simulink model "APFC_FullModel_v21b_Qmeas"  (R2025b)
settings: Solver=ode23t  StartTime=0.0  StopTime=50  MaxStep=2e-4  RelTol=1e-3
undefined symbols (not defined in the file): a_dq, ALPF_FAP_a, ALPF_FAP_b, ALPF_fine_alpha_delta, ALPF_fs, ALPF_gross_alpha, ALPF_k_powerOn, ALPF_LPF_g, ALPF_LPF_mag50_lin, ALPF_LPF_sos, ALPF_offset_inc_fine, ALPF_offset_inc_gross, b_dq, C_B1, C_B2, C_B3, DiscIntNeverNeededParam, dspblkCoreblockFVToolHelper, FLC_deadband_kVAR, gcbh, L_B1, L_B2, L_B3, omega, p, Q_reactor, Rc, tau_Qload, X1
libraries: ee_lib x63, fl_lib x59, nesl_utility x43, simulink x18, dspswit3 x9, dsparch4 x3, eeTransforms x2, fuzblock x1, eeSinusoidalMeasurementV2 x1
(part 2 of 5)

== system APFC_FullModel_v21b_Qmeas/ALPF2/CTRL ==
  IN : Inport
  YOUT : Inport  Port=2
  FSM : Subsystem  mask(ALPF CTRL FSM){}
      mask help:
      | ALPF CTRL FSM (Dossi US 12,294,375 B2, block 24). Parallel (AND) Stateflow
      | decomposition: phase branch ST0/ST1/ST2 on DIST, offset branch ST0/ST3/ST4 on
      | DISTORT, concurrent and independent. Three-threshold hysteresis per branch:
      | leave lock at |metric|>9, return at <3, escalate to gross at >21.
      | Phase: gross steps index by DIR and reads alpha = ALPF_gross_alpha(index); fine
      | accumulates alpha += ALPF_fine_alpha_delta(index)*DIR at the frozen index.
      | Offset: accumulates ADJ_offset by ALPF_offset_inc_fine (ST3) / ALPF_offset_inc_gross
      | (ST4), times the per-cycle OFFSET. Power-on index = ALPF_k_powerOn (40).
      | Reads ALPF_gross_alpha, ALPF_fine_alpha_delta, ALPF_k_powerOn, ALPF_offset_inc_fine,
      | ALPF_offset_inc_gross from the base workspace (APFC_Parameters.m). Double precision. Built and verified in four prove-then-mask stages. Documentation-only mask.
  OffsetBuffer : Subsystem  TreatAsAtomicUnit=on  mask(ALPF Phase Buffer){N=45}
      mask prompts: N "Buffer length N"
      mask help: FIFO of the most recent N=45 OFFSET values, clocked once per cycle by DZC; DISTORT = sum of buffer = distortion/offset metric, range −45…+45.
  PhaseBuffer : Subsystem  TreatAsAtomicUnit=on  mask(ALPF Phase Buffer){N=45}
      mask prompts: N "Buffer length N"
      mask help: FIFO of the most recent N=45 DIR values, clocked once per cycle by DZC; DIST = sum of buffer = phase‑mismatch metric, range −45…+45.
  SlopeDetector : Subsystem  mask(ALPF Slope Detector){}
      mask help: Computes SLOPE = |Slope_IN − Slope_YOUT| for the ALPF zero-crossing detector's adaptive threshold RESOL_THRES = MAX(IN)/4096 + SLOPE/4. Each per-sample slope (backward difference) is sampled and held at its own positive-going zero crossing. The absolute value guarantees SLOPE ≥ 0 so RESOL_THRES never falls below its MAX(IN)/4096 floor. Per Dossi patent (US 12,294,375 B2), block 21. SLOPE in per-sample units.
  ZCD : Subsystem  mask(ALPF Zero-Crossing Detector){}
      mask help: Computes zc=(IN+YOUT)/2; detects positive-going crossings of IN and YOUT; latches INC at YOUT's crossing and decodes DIR=INC−DEC, OFFSET=1−INC−DEC at IN's crossing (cycle boundary). RESOL_THRES = MAX(IN)/4096 + SLOPE/4.
  alpha : Outport
  index : Outport  Port=2
  ADJ_offset : Outport  Port=3
  SLOPE : Outport  Port=4
  DIR : Outport  Port=5
  DIST : Outport  Port=6
  OFFSET : Outport  Port=7
  DISTORT : Outport  Port=8
  wires:
  FSM/2(index) -> index/1
  ZCD/2(OFFSET) -> FSM/5(OFFSET), OFFSET/1, OffsetBuffer/1(OFFSET)  "OFFSET"
  ZCD/3(DZC) -> FSM/1(DZC), PhaseBuffer/Trigger, OffsetBuffer/Trigger
  IN/1 -> ZCD/1(IN), SlopeDetector/1(IN)
  YOUT/1 -> SlopeDetector/2(YOUT), ZCD/2(YOUT)
  ZCD/1(DIR) -> DIR/1, FSM/4(DIR), PhaseBuffer/1(DIR)  "DIR"
  SlopeDetector/1(SLOPE) -> SLOPE/1, ZCD/3(SLOPE)  "SLOPE"
  OffsetBuffer/1(DISTORT) -> FSM/3(DISTORT), DISTORT/1  "DISTORT"
  PhaseBuffer/1(DIST) -> DIST/1, FSM/2(DIST)  "DIST"
  FSM/1(alpha) -> alpha/1
  FSM/3(ADJ_offset) -> ADJ_offset/1

== system APFC_FullModel_v21b_Qmeas/ALPF2/FAP ==
  LPF_OUT : Inport
  Discrete Filter : DiscreteFilter  LoadFcn=dspblkCoreblockFVToolHelper(gcbh,'load');  Numerator=ALPF_FAP_b  Denominator=ALPF_FAP_a  FilterStructure=Direct form II transposed  a0EqualsOne=on
      settings: CopyFcn=dspblkCoreblockFVToolHelper(gcbh,'copy');  DeleteFcn=dspblkCoreblockFVToolHelper(gcbh,'close');  ModelCloseFcn=dspblkCoreblockFVToolHelper(gcbh,'close');  PreSaveFcn=dspblkCoreblockFVToolHelper(gcbh,'presave');  PostSaveFcn=dspblkCoreblockFVToolHelper(gcbh,'postsave');  CloseFcn=dspblkCoreblockFVToolHelper(gcbh,'close');
  FAP_OUT : Outport
  wires:
  LPF_OUT/1 -> Discrete Filter/1
  Discrete Filter/1 -> FAP_OUT/1

== system APFC_FullModel_v21b_Qmeas/ALPF2/LPF ==
  IN : Inport
  Biquad Filter : dsparch4/Biquad Filter  FilterSource=Dialog parameters  CoeffSource=Specify via dialog  FilterObject=BQF  IIRFiltStruct=Direct form II transposed  BiQuadCoeffs=ALPF_LPF_sos  ScaleValues=ALPF_LPF_g  IC=0  ICnum=0  ICden=0  a0Flag=Error  optimizeScaleValues=on  ScaleValueMode=Specify via input port (g)  roundingMode=Floor  overflowMode=off  scaleValueFracLength=14  denProdOutputFracLength=30  denAccumFracLength=30  secondMemoryFracLength=15
  LPF_OUT : Outport
  wires:
  Biquad Filter/1 -> LPF_OUT/1
  IN/1 -> Biquad Filter/1

== system APFC_FullModel_v21b_Qmeas/TSC Compensator/Bank_1 (5 kVAR) ==
  Enable_B1 : Inport
  TSC Bank 1 : Subsystem
      mask help:
      | Three-phase delta-connected TSC bank subsystem.
      | Contains three identical Delta_Limb instances (AB, BC, CA) and three line-to-line voltage sensors.
      |
      | Parameters C_val, L_val, and Rd_val are passed to all three Delta_Limb instances.
      | Default values correspond to Bank 1 (5 kVAR) at 415 V / 50 Hz with 6% detuning factor.
      |
      | Electrical ports: Phase_A, Phase_B, Phase_C.
      | Simulink inports: Gate_Drive_AB, Gate_Drive_BC, Gate_Drive_CA.
      | Simulink outports: V_AB, V_BC, V_CA (line voltages),
      | V_C0_AB, V_C0_BC, V_C0_CA (capacitor voltages),
      | V_sw_AB, V_sw_BC, V_sw_CA (thyristor switching voltages) are accessible via internal Scope blocks inside this subsystem.
      |
      | ZCD logic and Enable signals are external to this subsystem.
  ZCD Bank 1 : Subsystem
      mask help:
      | ZCD_Bank subsystem for one three-phase delta-connected TSC bank.
      | Contains ZCD_AB, ZCD_BC, ZCD_CA — one per delta limb.
      |
      | Inports: V_AB, V_BC, V_CA (line voltages from TSC_Bank),
      | V_C0_AB, V_C0_BC, V_C0_CA (capacitor voltages from TSC_Bank),
      | Enable (single switching command, broadcast to all three ZCDs).
      |
      | Outports: Gate_Drive_AB, Gate_Drive_BC, Gate_Drive_CA.
      |
      | One instance required per bank: ZCD_Bank_B1, ZCD_Bank_B2,
      | ZCD_Bank_B3.
  Phase_A : PMIOPort  Side=Left
  Phase_B : PMIOPort  Port=2  Side=Left
  Phase_C : PMIOPort  Port=3  Side=Left
  wires:
  TSC Bank 1/5(V_CA) -> ZCD Bank 1/5(V_CA)  "V_CA_B1"
  TSC Bank 1/2(V_CO_AB) -> ZCD Bank 1/2(V_CO_AB)  "V_CO_AB_B1"
  Enable_B1/1 -> ZCD Bank 1/7(Enable)
  TSC Bank 1/3(V_BC) -> ZCD Bank 1/3(V_BC)  "V_BC_B1"
  TSC Bank 1/1(V_AB) -> ZCD Bank 1/1(V_AB)  "V_AB_B1"
  TSC Bank 1/6(V_CO_CA) -> ZCD Bank 1/6(V_CO_CA)  "V_CO_CA_B1"
  TSC Bank 1/4(V_CO_BC) -> ZCD Bank 1/4(V_CO_BC)  "V_CO_BC_B1"
  ZCD Bank 1/1(Gate_drive_AB) -> TSC Bank 1/1(Gate_Drive_AB)
  ZCD Bank 1/2(Gate_drive_BC) -> TSC Bank 1/2(Gate_Drive_BC)
  ZCD Bank 1/3(Gate_drive_CA) -> TSC Bank 1/3(Gate_Drive_CA)
  connections:
  TSC Bank 1/LConn2 -- Phase_B/RConn1
  TSC Bank 1/LConn3 -- Phase_C/RConn1
  TSC Bank 1/LConn1 -- Phase_A/RConn1

== system APFC_FullModel_v21b_Qmeas/TSC Compensator/Bank_2 (10 kVAR) ==
  Enable_B2 : Inport
  TSC Bank 2 : Subsystem
      mask help:
      | Three-phase delta-connected TSC bank subsystem.
      | Contains three identical Delta_Limb instances (AB, BC, CA) and three line-to-line voltage sensors.
      |
      | Parameters C_val, L_val, and Rd_val are passed to all three Delta_Limb instances.
      | Default values correspond to Bank 2 (10 kVAR) at 415 V / 50 Hz with 6% detuning factor.
      |
      | Electrical ports: Phase_A, Phase_B, Phase_C.
      | Simulink inports: Gate_Drive_AB, Gate_Drive_BC, Gate_Drive_CA.
      | Simulink outports: V_AB, V_BC, V_CA (line voltages),
      | V_C0_AB, V_C0_BC, V_C0_CA (capacitor voltages),
      | V_sw_AB, V_sw_BC, V_sw_CA (thyristor switching voltages) are accessible via internal Scope blocks inside this subsystem.
      |
      | ZCD logic and Enable signals are external to this subsystem.
  ZCD Bank 2 : Subsystem
      mask help:
      | ZCD_Bank subsystem for one three-phase delta-connected TSC bank.
      | Contains ZCD_AB, ZCD_BC, ZCD_CA — one per delta limb.
      |
      | Inports: V_AB, V_BC, V_CA (line voltages from TSC_Bank),
      | V_C0_AB, V_C0_BC, V_C0_CA (capacitor voltages from TSC_Bank),
      | Enable (single switching command, broadcast to all three ZCDs).
      |
      | Outports: Gate_Drive_AB, Gate_Drive_BC, Gate_Drive_CA.
      |
      | One instance required per bank: ZCD_Bank_B1, ZCD_Bank_B2,
      | ZCD_Bank_B3.
  Phase_A : PMIOPort  Side=Left
  Phase_B : PMIOPort  Port=2  Side=Left
  Phase_C : PMIOPort  Port=3  Side=Left
  wires:
  TSC Bank 2/2(V_CO_AB) -> ZCD Bank 2/2(V_CO_AB)  "V_CO_AB_B2"
  TSC Bank 2/6(V_CO_CA) -> ZCD Bank 2/6(V_CO_CA)  "V_CO_CA_B2"
  TSC Bank 2/3(V_BC) -> ZCD Bank 2/3(V_BC)  "V_BC_B2"
  TSC Bank 2/5(V_CA) -> ZCD Bank 2/5(V_CA)  "V_CA_B2"
  TSC Bank 2/1(V_AB) -> ZCD Bank 2/1(V_AB)  "V_AB_B2"
  TSC Bank 2/4(V_CO_BC) -> ZCD Bank 2/4(V_CO_BC)  "V_CO_BC_B2"
  Enable_B2/1 -> ZCD Bank 2/7(Enable)
  ZCD Bank 2/1(Gate_drive_AB) -> TSC Bank 2/1(Gate_Drive_AB)
  ZCD Bank 2/2(Gate_drive_BC) -> TSC Bank 2/2(Gate_Drive_BC)
  ZCD Bank 2/3(Gate_drive_CA) -> TSC Bank 2/3(Gate_Drive_CA)
  connections:
  TSC Bank 2/LConn1 -- Phase_A/RConn1
  TSC Bank 2/LConn2 -- Phase_B/RConn1
  TSC Bank 2/LConn3 -- Phase_C/RConn1

== system APFC_FullModel_v21b_Qmeas/TSC Compensator/Bank_3 (20 kVAR) ==
  Enable_B3 : Inport
  TSC Bank 3 : Subsystem
      mask help:
      | Three-phase delta-connected TSC bank subsystem.
      | Contains three identical Delta_Limb instances (AB, BC, CA) and three line-to-line voltage sensors.
      |
      | Parameters C_val, L_val, and Rd_val are passed to all three Delta_Limb instances.
      | Default values correspond to Bank 3 (20 kVAR) at 415 V / 50 Hz with 6% detuning factor.
      |
      | Electrical ports: Phase_A, Phase_B, Phase_C.
      | Simulink inports: Gate_Drive_AB, Gate_Drive_BC, Gate_Drive_CA.
      | Simulink outports: V_AB, V_BC, V_CA (line voltages),
      | V_C0_AB, V_C0_BC, V_C0_CA (capacitor voltages),
      | V_sw_AB, V_sw_BC, V_sw_CA (thyristor switching voltages) are accessible via internal Scope blocks inside this subsystem.
      |
      | ZCD logic and Enable signals are external to this subsystem.
  ZCD Bank 3 : Subsystem
      mask help:
      | ZCD_Bank subsystem for one three-phase delta-connected TSC bank.
      | Contains ZCD_AB, ZCD_BC, ZCD_CA — one per delta limb.
      |
      | Inports: V_AB, V_BC, V_CA (line voltages from TSC_Bank),
      | V_C0_AB, V_C0_BC, V_C0_CA (capacitor voltages from TSC_Bank),
      | Enable (single switching command, broadcast to all three ZCDs).
      |
      | Outports: Gate_Drive_AB, Gate_Drive_BC, Gate_Drive_CA.
      |
      | One instance required per bank: ZCD_Bank_B1, ZCD_Bank_B2,
      | ZCD_Bank_B3.
  Phase_A : PMIOPort  Side=Left
  Phase_B : PMIOPort  Port=2  Side=Left
  Phase_C : PMIOPort  Port=3  Side=Left
  wires:
  TSC Bank 3/3(V_BC) -> ZCD Bank 3/3(V_BC)  "V_BC_B3"
  TSC Bank 3/4(V_CO_BC) -> ZCD Bank 3/4(V_CO_BC)  "V_CO_BC_B3"
  TSC Bank 3/6(V_CO_CA) -> ZCD Bank 3/6(V_CO_CA)  "V_CO_CA_B3"
  TSC Bank 3/5(V_CA) -> ZCD Bank 3/5(V_CA)  "V_CA_B3"
  TSC Bank 3/2(V_CO_AB) -> ZCD Bank 3/2(V_CO_AB)  "V_CO_AB_B3"
  TSC Bank 3/1(V_AB) -> ZCD Bank 3/1(V_AB)  "V_AB_B3"
  Enable_B3/1 -> ZCD Bank 3/7(Enable)
  ZCD Bank 3/1(Gate_drive_AB) -> TSC Bank 3/1(Gate_Drive_AB)
  ZCD Bank 3/2(Gate_drive_BC) -> TSC Bank 3/2(Gate_Drive_BC)
  ZCD Bank 3/3(Gate_drive_CA) -> TSC Bank 3/3(Gate_Drive_CA)
  connections:
  Phase_B/RConn1 -- TSC Bank 3/LConn2
  Phase_A/RConn1 -- TSC Bank 3/LConn1
  Phase_C/RConn1 -- TSC Bank 3/LConn3

== system APFC_FullModel_v21b_Qmeas/ALPF/CTRL/FSM ==
  DZC : Inport
  DIST : Inport  Port=2
  DISTORT : Inport  Port=3
  DIR : Inport  Port=4
  OFFSET : Inport  Port=5
  ALPF_FSM : Stateflow chart  TreatAsAtomicUnit=on
  alpha : Outport
  index : Outport  Port=2
  ADJ_offset : Outport  Port=3
  wires:
  ALPF_FSM/2(index) -> index/1
  DZC/1 -> ALPF_FSM/Trigger
  OFFSET/1 -> ALPF_FSM/4(OFFSET)
  ALPF_FSM/1(alpha) -> alpha/1
  DISTORT/1 -> ALPF_FSM/2(DISTORT)
  ALPF_FSM/3(ADJ_offset) -> ADJ_offset/1
  DIST/1 -> ALPF_FSM/1(DIST)
  DIR/1 -> ALPF_FSM/3(DIR)

== system APFC_FullModel_v21b_Qmeas/ALPF/CTRL/OffsetBuffer ==
  OFFSET : Inport
  Trigger : TriggerPort  VariantControl=(inherit)
  Sum of Elements : Sum  Inputs=+
  Tapped Delay : simulink/Discrete/Tapped Delay  vinit=0.0  samptime=-1  NumDelays=N-1  DelayOrder=Oldest  includeCurrent=on
  DISTORT : Outport
  wires:
  OFFSET/1 -> Tapped Delay/1
  Tapped Delay/1 -> Sum of Elements/1
  Sum of Elements/1 -> DISTORT/1

== system APFC_FullModel_v21b_Qmeas/ALPF/CTRL/PhaseBuffer ==
  DIR : Inport
  Trigger : TriggerPort  VariantControl=(inherit)
  Sum of Elements : Sum  Inputs=+
  Tapped Delay : simulink/Discrete/Tapped Delay  vinit=0.0  samptime=-1  NumDelays=N-1  DelayOrder=Oldest  includeCurrent=on
  DIST : Outport
  wires:
  DIR/1 -> Tapped Delay/1
  Tapped Delay/1 -> Sum of Elements/1
  Sum of Elements/1 -> DIST/1

== system APFC_FullModel_v21b_Qmeas/ALPF/CTRL/SlopeDetector ==
  IN : Inport
  YOUT : Inport  Port=2
  Abs : Abs  SaturateOnIntegerOverflow=off
  Detect Rise Nonnegative : simulink/Logic and Bit Operations/Detect Rise Nonnegative  vinit=0  OutDataTypeStr=boolean
  Detect Rise Nonnegative1 : simulink/Logic and Bit Operations/Detect Rise Nonnegative  vinit=0  OutDataTypeStr=boolean
  Hold_SlopeIN : Subsystem  TreatAsAtomicUnit=on
  Hold_SlopeYOUT : Subsystem  TreatAsAtomicUnit=on
  Subtract : Sum  Inputs=+-
  Subtract1 : Sum  Inputs=+-
  Subtract2 : Sum  Inputs=+-
  Unit Delay : UnitDelay  SampleTime=1/12500  HasFrameUpgradeWarning=on
  Unit Delay1 : UnitDelay  SampleTime=1/12500  HasFrameUpgradeWarning=on
  SLOPE : Outport
  wires:
  Subtract2/1 -> Abs/1  "Slope_diff"
  Abs/1 -> SLOPE/1  "SLOPE"
  Hold_SlopeYOUT/1(Out1) -> Subtract2/2  "Slope_YOUT_held"
  YOUT/1 -> Detect Rise Nonnegative1/1, Unit Delay1/1, Subtract1/1
  Detect Rise Nonnegative/1 -> Hold_SlopeIN/Trigger  "IN_posZC"
  Subtract/1 -> Hold_SlopeIN/1(In1)  "Slope_IN"
  Unit Delay1/1 -> Subtract1/2
  Detect Rise Nonnegative1/1 -> Hold_SlopeYOUT/Trigger  "YOUT_posZC"
  IN/1 -> Unit Delay/1, Detect Rise Nonnegative/1, Subtract/1
  Subtract1/1 -> Hold_SlopeYOUT/1(In1)  "Slope_YOUT"
  Hold_SlopeIN/1(Out1) -> Subtract2/1  "Slope_IN_held"
  Unit Delay/1 -> Subtract/2

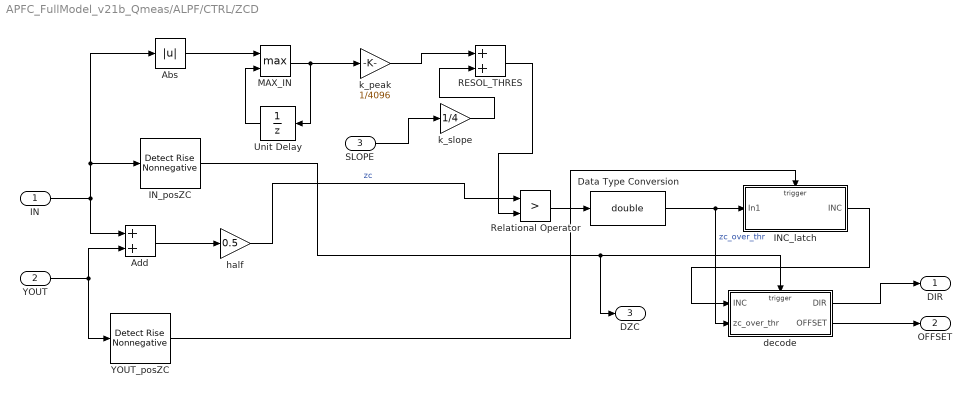
== system APFC_FullModel_v21b_Qmeas/ALPF/CTRL/ZCD ==
  IN : Inport
  YOUT : Inport  Port=2
  SLOPE : Inport  Port=3
  Abs : Abs  SaturateOnIntegerOverflow=off
  Add : Sum
  Data Type Conversion : DataTypeConversion  OutDataTypeStr=double  SaturateOnIntegerOverflow=off  RndMeth=Floor
  INC_latch : Subsystem  TreatAsAtomicUnit=on
  IN_posZC : simulink/Logic and Bit Operations/Detect Rise Nonnegative  vinit=0  OutDataTypeStr=boolean
  MAX_IN : MinMax  Function=max  Inputs=2
  RESOL_THRES : Sum
  Relational Operator : RelationalOperator  Operator=>  OutDataTypeStr=boolean  RndMeth=Simplest  InputSameDT=off
  Unit Delay : UnitDelay  SampleTime=1/12500  HasFrameUpgradeWarning=on
  YOUT_posZC : simulink/Logic and Bit Operations/Detect Rise Nonnegative  vinit=0  OutDataTypeStr=boolean
  decode : Subsystem  TreatAsAtomicUnit=on
  half : Gain  Gain=0.5
  k_peak : Gain  Gain=1/4096
  k_slope : Gain  Gain=1/4
  DIR : Outport
  OFFSET : Outport  Port=2
  DZC : Outport  Port=3
  wires:
  Data Type Conversion/1 -> decode/2(zc_over_thr), INC_latch/1(In1)  "zc_over_thr"
  half/1 -> Relational Operator/1  "zc"
  Relational Operator/1 -> Data Type Conversion/1
  SLOPE/1 -> k_slope/1
  YOUT/1 -> YOUT_posZC/1, Add/2
  RESOL_THRES/1 -> Relational Operator/2
  Add/1 -> half/1
  decode/1(DIR) -> DIR/1
  IN/1 -> IN_posZC/1, Abs/1, Add/1
  YOUT_posZC/1 -> INC_latch/Trigger
  MAX_IN/1 -> Unit Delay/1, k_peak/1
  IN_posZC/1 -> DZC/1, decode/Trigger
  INC_latch/1(INC) -> decode/1(INC)
  Unit Delay/1 -> MAX_IN/2
  Abs/1 -> MAX_IN/1
  k_slope/1 -> RESOL_THRES/2
  decode/2(OFFSET) -> OFFSET/1
  k_peak/1 -> RESOL_THRES/1

== system APFC_FullModel_v21b_Qmeas/ALPF1/CTRL/FSM ==
  DZC : Inport
  DIST : Inport  Port=2
  DISTORT : Inport  Port=3
  DIR : Inport  Port=4
  OFFSET : Inport  Port=5
  ALPF_FSM : Stateflow chart  TreatAsAtomicUnit=on
  alpha : Outport
  index : Outport  Port=2
  ADJ_offset : Outport  Port=3
  wires:
  ALPF_FSM/2(index) -> index/1
  DZC/1 -> ALPF_FSM/Trigger
  OFFSET/1 -> ALPF_FSM/4(OFFSET)
  ALPF_FSM/1(alpha) -> alpha/1
  DISTORT/1 -> ALPF_FSM/2(DISTORT)
  ALPF_FSM/3(ADJ_offset) -> ADJ_offset/1
  DIST/1 -> ALPF_FSM/1(DIST)
  DIR/1 -> ALPF_FSM/3(DIR)

== system APFC_FullModel_v21b_Qmeas/ALPF1/CTRL/OffsetBuffer ==
  OFFSET : Inport
  Trigger : TriggerPort  VariantControl=(inherit)
  Sum of Elements : Sum  Inputs=+
  Tapped Delay : simulink/Discrete/Tapped Delay  vinit=0.0  samptime=-1  NumDelays=N-1  DelayOrder=Oldest  includeCurrent=on
  DISTORT : Outport
  wires:
  OFFSET/1 -> Tapped Delay/1
  Tapped Delay/1 -> Sum of Elements/1
  Sum of Elements/1 -> DISTORT/1

== system APFC_FullModel_v21b_Qmeas/ALPF1/CTRL/PhaseBuffer ==
  DIR : Inport
  Trigger : TriggerPort  VariantControl=(inherit)
  Sum of Elements : Sum  Inputs=+
  Tapped Delay : simulink/Discrete/Tapped Delay  vinit=0.0  samptime=-1  NumDelays=N-1  DelayOrder=Oldest  includeCurrent=on
  DIST : Outport
  wires:
  DIR/1 -> Tapped Delay/1
  Tapped Delay/1 -> Sum of Elements/1
  Sum of Elements/1 -> DIST/1

== system APFC_FullModel_v21b_Qmeas/ALPF1/CTRL/SlopeDetector ==
  IN : Inport
  YOUT : Inport  Port=2
  Abs : Abs  SaturateOnIntegerOverflow=off
  Detect Rise Nonnegative : simulink/Logic and Bit Operations/Detect Rise Nonnegative  vinit=0  OutDataTypeStr=boolean
  Detect Rise Nonnegative1 : simulink/Logic and Bit Operations/Detect Rise Nonnegative  vinit=0  OutDataTypeStr=boolean
  Hold_SlopeIN : Subsystem  TreatAsAtomicUnit=on
  Hold_SlopeYOUT : Subsystem  TreatAsAtomicUnit=on
  Subtract : Sum  Inputs=+-
  Subtract1 : Sum  Inputs=+-
  Subtract2 : Sum  Inputs=+-
  Unit Delay : UnitDelay  SampleTime=1/12500  HasFrameUpgradeWarning=on
  Unit Delay1 : UnitDelay  SampleTime=1/12500  HasFrameUpgradeWarning=on
  SLOPE : Outport
  wires:
  Subtract2/1 -> Abs/1  "Slope_diff"
  Abs/1 -> SLOPE/1  "SLOPE"
  Hold_SlopeYOUT/1(Out1) -> Subtract2/2  "Slope_YOUT_held"
  YOUT/1 -> Detect Rise Nonnegative1/1, Unit Delay1/1, Subtract1/1
  Detect Rise Nonnegative/1 -> Hold_SlopeIN/Trigger  "IN_posZC"
  Subtract/1 -> Hold_SlopeIN/1(In1)  "Slope_IN"
  Unit Delay1/1 -> Subtract1/2
  Detect Rise Nonnegative1/1 -> Hold_SlopeYOUT/Trigger  "YOUT_posZC"
  IN/1 -> Unit Delay/1, Detect Rise Nonnegative/1, Subtract/1
  Subtract1/1 -> Hold_SlopeYOUT/1(In1)  "Slope_YOUT"
  Hold_SlopeIN/1(Out1) -> Subtract2/1  "Slope_IN_held"
  Unit Delay/1 -> Subtract/2

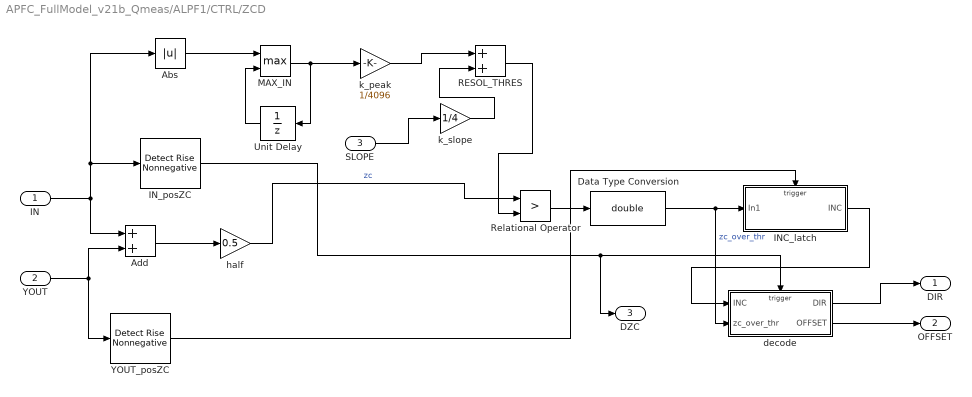
== system APFC_FullModel_v21b_Qmeas/ALPF1/CTRL/ZCD ==
  IN : Inport
  YOUT : Inport  Port=2
  SLOPE : Inport  Port=3
  Abs : Abs  SaturateOnIntegerOverflow=off
  Add : Sum
  Data Type Conversion : DataTypeConversion  OutDataTypeStr=double  SaturateOnIntegerOverflow=off  RndMeth=Floor
  INC_latch : Subsystem  TreatAsAtomicUnit=on
  IN_posZC : simulink/Logic and Bit Operations/Detect Rise Nonnegative  vinit=0  OutDataTypeStr=boolean
  MAX_IN : MinMax  Function=max  Inputs=2
  RESOL_THRES : Sum
  Relational Operator : RelationalOperator  Operator=>  OutDataTypeStr=boolean  RndMeth=Simplest  InputSameDT=off
  Unit Delay : UnitDelay  SampleTime=1/12500  HasFrameUpgradeWarning=on
  YOUT_posZC : simulink/Logic and Bit Operations/Detect Rise Nonnegative  vinit=0  OutDataTypeStr=boolean
  decode : Subsystem  TreatAsAtomicUnit=on
  half : Gain  Gain=0.5
  k_peak : Gain  Gain=1/4096
  k_slope : Gain  Gain=1/4
  DIR : Outport
  OFFSET : Outport  Port=2
  DZC : Outport  Port=3
  wires:
  Data Type Conversion/1 -> decode/2(zc_over_thr), INC_latch/1(In1)  "zc_over_thr"
  half/1 -> Relational Operator/1  "zc"
  Relational Operator/1 -> Data Type Conversion/1
  SLOPE/1 -> k_slope/1
  YOUT/1 -> YOUT_posZC/1, Add/2
  RESOL_THRES/1 -> Relational Operator/2
  Add/1 -> half/1
  decode/1(DIR) -> DIR/1
  IN/1 -> IN_posZC/1, Abs/1, Add/1
  YOUT_posZC/1 -> INC_latch/Trigger
  MAX_IN/1 -> Unit Delay/1, k_peak/1
  IN_posZC/1 -> DZC/1, decode/Trigger
  INC_latch/1(INC) -> decode/1(INC)
  Unit Delay/1 -> MAX_IN/2
  Abs/1 -> MAX_IN/1
  k_slope/1 -> RESOL_THRES/2
  decode/2(OFFSET) -> OFFSET/1
  k_peak/1 -> RESOL_THRES/1

== system APFC_FullModel_v21b_Qmeas/ALPF2/CTRL/FSM ==
  DZC : Inport
  DIST : Inport  Port=2
  DISTORT : Inport  Port=3
  DIR : Inport  Port=4
  OFFSET : Inport  Port=5
  ALPF_FSM : Stateflow chart  TreatAsAtomicUnit=on
  alpha : Outport
  index : Outport  Port=2
  ADJ_offset : Outport  Port=3
  wires:
  ALPF_FSM/2(index) -> index/1
  DZC/1 -> ALPF_FSM/Trigger
  OFFSET/1 -> ALPF_FSM/4(OFFSET)
  ALPF_FSM/1(alpha) -> alpha/1
  DISTORT/1 -> ALPF_FSM/2(DISTORT)
  ALPF_FSM/3(ADJ_offset) -> ADJ_offset/1
  DIST/1 -> ALPF_FSM/1(DIST)
  DIR/1 -> ALPF_FSM/3(DIR)

== system APFC_FullModel_v21b_Qmeas/ALPF2/CTRL/OffsetBuffer ==
  OFFSET : Inport
  Trigger : TriggerPort  VariantControl=(inherit)
  Sum of Elements : Sum  Inputs=+
  Tapped Delay : simulink/Discrete/Tapped Delay  vinit=0.0  samptime=-1  NumDelays=N-1  DelayOrder=Oldest  includeCurrent=on
  DISTORT : Outport
  wires:
  OFFSET/1 -> Tapped Delay/1
  Tapped Delay/1 -> Sum of Elements/1
  Sum of Elements/1 -> DISTORT/1

== system APFC_FullModel_v21b_Qmeas/ALPF2/CTRL/PhaseBuffer ==
  DIR : Inport
  Trigger : TriggerPort  VariantControl=(inherit)
  Sum of Elements : Sum  Inputs=+
  Tapped Delay : simulink/Discrete/Tapped Delay  vinit=0.0  samptime=-1  NumDelays=N-1  DelayOrder=Oldest  includeCurrent=on
  DIST : Outport
  wires:
  DIR/1 -> Tapped Delay/1
  Tapped Delay/1 -> Sum of Elements/1
  Sum of Elements/1 -> DIST/1

== system APFC_FullModel_v21b_Qmeas/ALPF2/CTRL/SlopeDetector ==
  IN : Inport
  YOUT : Inport  Port=2
  Abs : Abs  SaturateOnIntegerOverflow=off
  Detect Rise Nonnegative : simulink/Logic and Bit Operations/Detect Rise Nonnegative  vinit=0  OutDataTypeStr=boolean
  Detect Rise Nonnegative1 : simulink/Logic and Bit Operations/Detect Rise Nonnegative  vinit=0  OutDataTypeStr=boolean
  Hold_SlopeIN : Subsystem  TreatAsAtomicUnit=on
  Hold_SlopeYOUT : Subsystem  TreatAsAtomicUnit=on
  Subtract : Sum  Inputs=+-
  Subtract1 : Sum  Inputs=+-
  Subtract2 : Sum  Inputs=+-
  Unit Delay : UnitDelay  SampleTime=1/12500  HasFrameUpgradeWarning=on
  Unit Delay1 : UnitDelay  SampleTime=1/12500  HasFrameUpgradeWarning=on
  SLOPE : Outport
  wires:
  Subtract2/1 -> Abs/1  "Slope_diff"
  Abs/1 -> SLOPE/1  "SLOPE"
  Hold_SlopeYOUT/1(Out1) -> Subtract2/2  "Slope_YOUT_held"
  YOUT/1 -> Detect Rise Nonnegative1/1, Unit Delay1/1, Subtract1/1
  Detect Rise Nonnegative/1 -> Hold_SlopeIN/Trigger  "IN_posZC"
  Subtract/1 -> Hold_SlopeIN/1(In1)  "Slope_IN"
  Unit Delay1/1 -> Subtract1/2
  Detect Rise Nonnegative1/1 -> Hold_SlopeYOUT/Trigger  "YOUT_posZC"
  IN/1 -> Unit Delay/1, Detect Rise Nonnegative/1, Subtract/1
  Subtract1/1 -> Hold_SlopeYOUT/1(In1)  "Slope_YOUT"
  Hold_SlopeIN/1(Out1) -> Subtract2/1  "Slope_IN_held"
  Unit Delay/1 -> Subtract/2

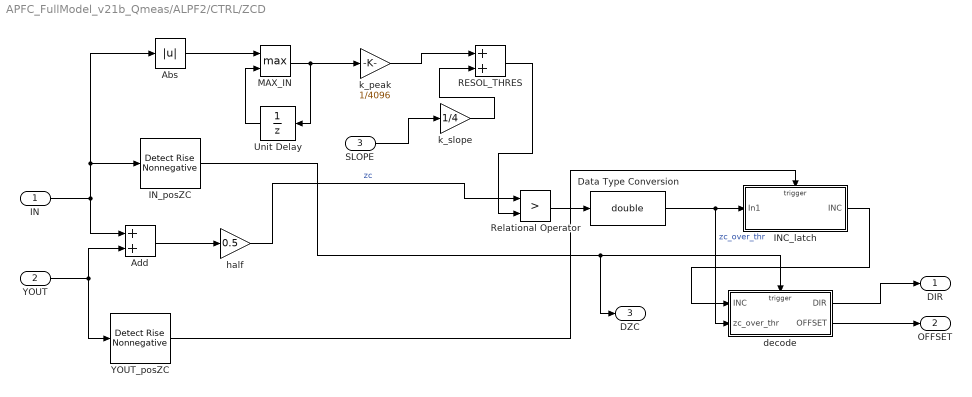
== system APFC_FullModel_v21b_Qmeas/ALPF2/CTRL/ZCD ==
  IN : Inport
  YOUT : Inport  Port=2
  SLOPE : Inport  Port=3
  Abs : Abs  SaturateOnIntegerOverflow=off
  Add : Sum
  Data Type Conversion : DataTypeConversion  OutDataTypeStr=double  SaturateOnIntegerOverflow=off  RndMeth=Floor
  INC_latch : Subsystem  TreatAsAtomicUnit=on
  IN_posZC : simulink/Logic and Bit Operations/Detect Rise Nonnegative  vinit=0  OutDataTypeStr=boolean
  MAX_IN : MinMax  Function=max  Inputs=2
  RESOL_THRES : Sum
  Relational Operator : RelationalOperator  Operator=>  OutDataTypeStr=boolean  RndMeth=Simplest  InputSameDT=off
  Unit Delay : UnitDelay  SampleTime=1/12500  HasFrameUpgradeWarning=on
  YOUT_posZC : simulink/Logic and Bit Operations/Detect Rise Nonnegative  vinit=0  OutDataTypeStr=boolean
  decode : Subsystem  TreatAsAtomicUnit=on
  half : Gain  Gain=0.5
  k_peak : Gain  Gain=1/4096
  k_slope : Gain  Gain=1/4
  DIR : Outport
  OFFSET : Outport  Port=2
  DZC : Outport  Port=3
  wires:
  Data Type Conversion/1 -> decode/2(zc_over_thr), INC_latch/1(In1)  "zc_over_thr"
  half/1 -> Relational Operator/1  "zc"
  Relational Operator/1 -> Data Type Conversion/1
  SLOPE/1 -> k_slope/1
  YOUT/1 -> YOUT_posZC/1, Add/2
  RESOL_THRES/1 -> Relational Operator/2
  Add/1 -> half/1
  decode/1(DIR) -> DIR/1
  IN/1 -> IN_posZC/1, Abs/1, Add/1
  YOUT_posZC/1 -> INC_latch/Trigger
  MAX_IN/1 -> Unit Delay/1, k_peak/1
  IN_posZC/1 -> DZC/1, decode/Trigger
  INC_latch/1(INC) -> decode/1(INC)
  Unit Delay/1 -> MAX_IN/2
  Abs/1 -> MAX_IN/1
  k_slope/1 -> RESOL_THRES/2
  decode/2(OFFSET) -> OFFSET/1
  k_peak/1 -> RESOL_THRES/1

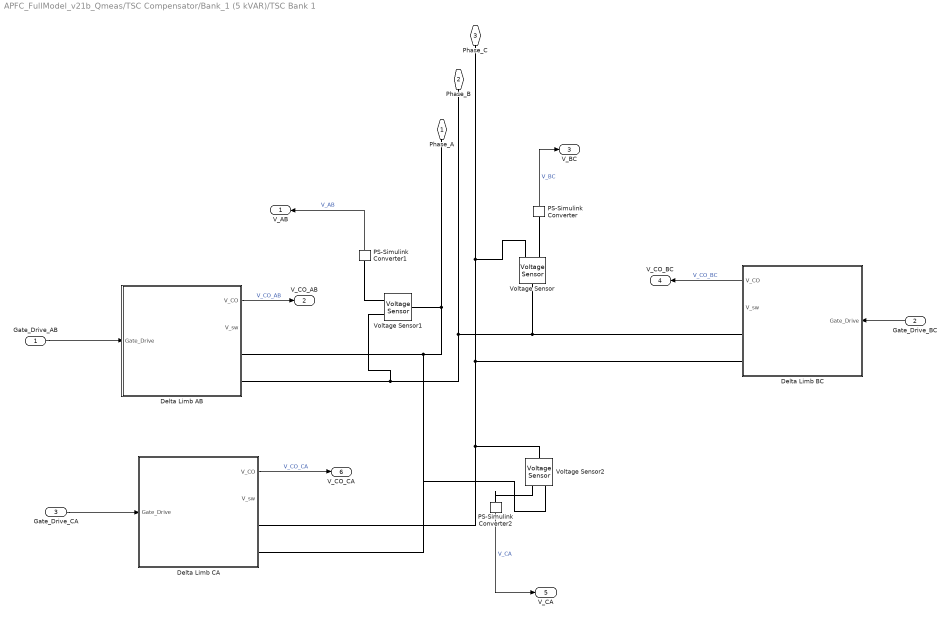
== system APFC_FullModel_v21b_Qmeas/TSC Compensator/Bank_1 (5 kVAR)/TSC Bank 1 ==
  Gate_Drive_AB : Inport
  Gate_Drive_BC : Inport  Port=2
  Gate_Drive_CA : Inport  Port=3
  Delta Limb AB : Subsystem  mask{C_val=C_B1, L_val=L_B1, Rd_val=100e3}
      mask prompts: C_val "Capacitance (F)"; L_val "Inductance (H)"; Rd_val "Discharge Resistance (Ohm)"
      mask help:
      | Delta limb of a three-phase delta-connected TSC bank.
      | Contains: anti-parallel thyristor pair, detuning reactor (L_val,
      | R_series = omega*L_val/Q_reactor), shunt capacitor (C_val), parallel discharge
      | resistor (Rd_val), RC snubber (100 Ohm, 0.1 uF).
      |
      | Output signals:
      | V_sw: instantaneous voltage across the anti-parallel thyristor pair.
      | Used as a diagnostic signal to verify transient-free switching.
      | At the moment of firing, V_sw should be at or near zero. After
      | turn-off, V_sw reflects the difference between the line-to-line
      | source voltage and the capacitor voltage V_C0.
      |
      | V_C0: instantaneous voltage across the shunt capacitor. Fed
      | externally to the ZCD comparator as the residual capacitor voltage
      | reference for voltage-matched firing on subsequent switching events.
      |
      | ZCD logic and gate drive signals are external to this subsystem.
      | Default values correspond to Bank 3 (20 kVAR) at 415 V / 50 Hz
      | with 6% detuning factor. Parameter values for Bank 1 (5 kVAR) and
      | Bank 2 (10 kVAR) are assigned by editing the mask dialog at
      | instantiation.
  Delta Limb BC : Subsystem  mask{C_val=C_B1, L_val=L_B1, Rd_val=100e3}
      mask prompts: C_val "Capacitance (F)"; L_val "Inductance (H)"; Rd_val "Discharge Resistance (Ohm)"
      mask help:
      | Delta limb of a three-phase delta-connected TSC bank.
      | Contains: anti-parallel thyristor pair, detuning reactor (L_val,
      | R_series = omega*L_val/Q_reactor), shunt capacitor (C_val), parallel discharge
      | resistor (Rd_val), RC snubber (100 Ohm, 0.1 uF).
      |
      | Output signals:
      | V_sw: instantaneous voltage across the anti-parallel thyristor pair.
      | Used as a diagnostic signal to verify transient-free switching.
      | At the moment of firing, V_sw should be at or near zero. After
      | turn-off, V_sw reflects the difference between the line-to-line
      | source voltage and the capacitor voltage V_C0.
      |
      | V_C0: instantaneous voltage across the shunt capacitor. Fed
      | externally to the ZCD comparator as the residual capacitor voltage
      | reference for voltage-matched firing on subsequent switching events.
      |
      | ZCD logic and gate drive signals are external to this subsystem.
      | Default values correspond to Bank 3 (20 kVAR) at 415 V / 50 Hz
      | with 6% detuning factor. Parameter values for Bank 1 (5 kVAR) and
      | Bank 2 (10 kVAR) are assigned by editing the mask dialog at
      | instantiation.
  Delta Limb CA : Subsystem  mask{C_val=C_B1, L_val=L_B1, Rd_val=100e3}
      mask prompts: C_val "Capacitance (F)"; L_val "Inductance (H)"; Rd_val "Discharge Resistance (Ohm)"
      mask help:
      | Delta limb of a three-phase delta-connected TSC bank.
      | Contains: anti-parallel thyristor pair, detuning reactor (L_val,
      | R_series = omega*L_val/Q_reactor), shunt capacitor (C_val), parallel discharge
      | resistor (Rd_val), RC snubber (100 Ohm, 0.1 uF).
      |
      | Output signals:
      | V_sw: instantaneous voltage across the anti-parallel thyristor pair.
      | Used as a diagnostic signal to verify transient-free switching.
      | At the moment of firing, V_sw should be at or near zero. After
      | turn-off, V_sw reflects the difference between the line-to-line
      | source voltage and the capacitor voltage V_C0.
      |
      | V_C0: instantaneous voltage across the shunt capacitor. Fed
      | externally to the ZCD comparator as the residual capacitor voltage
      | reference for voltage-matched firing on subsequent switching events.
      |
      | ZCD logic and gate drive signals are external to this subsystem.
      | Default values correspond to Bank 3 (20 kVAR) at 415 V / 50 Hz
      | with 6% detuning factor. Parameter values for Bank 1 (5 kVAR) and
      | Bank 2 (10 kVAR) are assigned by editing the mask dialog at
      | instantiation.
  PS-Simulink Converter : nesl_utility/PS-Simulink Converter  PhysicalDomain=network_engine_domain  SubClassName=ps_output  LeftPortType=input  RightPortType=output  PseudoPeriodic=off  Frequencies=[]  VectorFormat=inherit  Unit=inherit  AffineConversion=off
  PS-Simulink Converter1 : nesl_utility/PS-Simulink Converter  PhysicalDomain=network_engine_domain  SubClassName=ps_output  LeftPortType=input  RightPortType=output  PseudoPeriodic=off  Frequencies=[]  VectorFormat=inherit  Unit=inherit  AffineConversion=off
  PS-Simulink Converter2 : nesl_utility/PS-Simulink Converter  PhysicalDomain=network_engine_domain  SubClassName=ps_output  LeftPortType=input  RightPortType=output  PseudoPeriodic=off  Frequencies=[]  VectorFormat=inherit  Unit=inherit  AffineConversion=off
  Voltage Sensor : fl_lib/Electrical/Electrical Sensors/Voltage Sensor
  Voltage Sensor1 : fl_lib/Electrical/Electrical Sensors/Voltage Sensor
  Voltage Sensor2 : fl_lib/Electrical/Electrical Sensors/Voltage Sensor
  Phase_A : PMIOPort  Side=Left
  Phase_B : PMIOPort  Port=2  Side=Left
  Phase_C : PMIOPort  Port=3  Side=Left
  V_AB : Outport
  V_CO_AB : Outport  Port=2
  V_BC : Outport  Port=3
  V_CO_BC : Outport  Port=4
  V_CA : Outport  Port=5
  V_CO_CA : Outport  Port=6
  wires:
  Delta Limb BC/1(V_CO) -> V_CO_BC/1  "V_CO_BC"
  PS-Simulink Converter/1 -> V_BC/1  "V_BC"
  Gate_Drive_CA/1 -> Delta Limb CA/1(Gate_Drive)
  PS-Simulink Converter1/1 -> V_AB/1  "V_AB"
  Delta Limb AB/1(V_CO) -> V_CO_AB/1  "V_CO_AB"
  Delta Limb CA/1(V_CO) -> V_CO_CA/1  "V_CO_CA"
  Gate_Drive_BC/1 -> Delta Limb BC/1(Gate_Drive)
  Gate_Drive_AB/1 -> Delta Limb AB/1(Gate_Drive)
  PS-Simulink Converter2/1 -> V_CA/1  "V_CA"
  connections:
  Delta Limb BC/RConn1 -- Voltage Sensor/LConn1 -- Phase_B/RConn1 -- Voltage Sensor1/RConn2 -- Delta Limb AB/RConn2
  Voltage Sensor1/RConn1 -- PS-Simulink Converter1/LConn1
  PS-Simulink Converter2/LConn1 -- Voltage Sensor2/RConn1
  Voltage Sensor/RConn2 -- Phase_C/RConn1 -- Delta Limb BC/RConn2 -- Voltage Sensor2/LConn1 -- Delta Limb CA/RConn1
  Voltage Sensor/RConn1 -- PS-Simulink Converter/LConn1
  Voltage Sensor1/LConn1 -- Phase_A/RConn1 -- Voltage Sensor2/RConn2 -- Delta Limb CA/RConn2 -- Delta Limb AB/RConn1

== system APFC_FullModel_v21b_Qmeas/TSC Compensator/Bank_1 (5 kVAR)/ZCD Bank 1 ==
  V_AB : Inport
  V_CO_AB : Inport  Port=2
  V_BC : Inport  Port=3
  V_CO_BC : Inport  Port=4
  V_CA : Inport  Port=5
  V_CO_CA : Inport  Port=6
  Enable : Inport  Port=7
  ZCD AB : Subsystem
      mask help:
      | Zero-Crossing Detection (ZCD) subsystem for one delta limb of a
      | three-phase delta-connected TSC bank.
      |
      | Implements voltage-matched firing logic for transient-free
      | thyristor switching.
      |
      | Inputs:
      | V_source: instantaneous line-to-line voltage for this limb,
      | fed through a Unit Delay (T_s = 0.0001 s) to the comparator.
      |
      | V_C0: residual capacitor voltage from the corresponding
      | Delta_Limb instance, fed through a Unit Delay (T_s = 0.0001 s)
      | to the comparator.
      |
      | Enable: FLC switching command (S = 1 to arm, S = 0 to inhibit).
      | Set to Constant = 1 for open-loop testing.
      |
      | Output:
      | Gate_drive: firing pulse issued when V_source >= V_C0 on a
      | rising edge, AND Enable = 1. Fed to the Gate_drive inport of
      | the corresponding Delta_Limb instance.
      |
      | Internal blocks: Unit Delay (x2), Relational Operator (>=),
      | Zero-Order Hold (T_s = 0.0001 s), Edge Detector (rising edge),
      | AND gate.
      |
      | One instance required per delta limb: ZCD_AB, ZCD_BC, ZCD_CA.
  ZCD BC : Subsystem
      mask help:
      | Zero-Crossing Detection (ZCD) subsystem for one delta limb of a
      | three-phase delta-connected TSC bank.
      |
      | Implements voltage-matched firing logic for transient-free
      | thyristor switching.
      |
      | Inputs:
      | V_source: instantaneous line-to-line voltage for this limb,
      | fed through a Unit Delay (T_s = 0.0001 s) to the comparator.
      |
      | V_C0: residual capacitor voltage from the corresponding
      | Delta_Limb instance, fed through a Unit Delay (T_s = 0.0001 s)
      | to the comparator.
      |
      | Enable: FLC switching command (S = 1 to arm, S = 0 to inhibit).
      | Set to Constant = 1 for open-loop testing.
      |
      | Output:
      | Gate_drive: firing pulse issued when V_source >= V_C0 on a
      | rising edge, AND Enable = 1. Fed to the Gate_drive inport of
      | the corresponding Delta_Limb instance.
      |
      | Internal blocks: Unit Delay (x2), Relational Operator (>=),
      | Zero-Order Hold (T_s = 0.0001 s), Edge Detector (rising edge),
      | AND gate.
      |
      | One instance required per delta limb: ZCD_AB, ZCD_BC, ZCD_CA.
  ZCD CA : Subsystem
      mask help:
      | Zero-Crossing Detection (ZCD) subsystem for one delta limb of a
      | three-phase delta-connected TSC bank.
      |
      | Implements voltage-matched firing logic for transient-free
      | thyristor switching.
      |
      | Inputs:
      | V_source: instantaneous line-to-line voltage for this limb,
      | fed through a Unit Delay (T_s = 0.0001 s) to the comparator.
      |
      | V_C0: residual capacitor voltage from the corresponding
      | Delta_Limb instance, fed through a Unit Delay (T_s = 0.0001 s)
      | to the comparator.
      |
      | Enable: FLC switching command (S = 1 to arm, S = 0 to inhibit).
      | Set to Constant = 1 for open-loop testing.
      |
      | Output:
      | Gate_drive: firing pulse issued when V_source >= V_C0 on a
      | rising edge, AND Enable = 1. Fed to the Gate_drive inport of
      | the corresponding Delta_Limb instance.
      |
      | Internal blocks: Unit Delay (x2), Relational Operator (>=),
      | Zero-Order Hold (T_s = 0.0001 s), Edge Detector (rising edge),
      | AND gate.
      |
      | One instance required per delta limb: ZCD_AB, ZCD_BC, ZCD_CA.
  Gate_drive_AB : Outport
  Gate_drive_BC : Outport  Port=2
  Gate_drive_CA : Outport  Port=3
  wires:
  V_BC/1 -> ZCD BC/2(V_BC)
  Enable/1 -> ZCD AB/3(Enable), ZCD CA/3(Enable), ZCD BC/3(Enable)
  V_CO_BC/1 -> ZCD BC/1(V_CO_BC)
  V_CA/1 -> ZCD CA/2(V_CA)
  V_AB/1 -> ZCD AB/2(V_AB)
  ZCD BC/1(Gate_drive_BC) -> Gate_drive_BC/1
  V_CO_CA/1 -> ZCD CA/1(V_CO_CA)
  ZCD AB/1(Gate_drive_AB) -> Gate_drive_AB/1
  V_CO_AB/1 -> ZCD AB/1(V_CO_AB)
  ZCD CA/1(Gate_drive_CA) -> Gate_drive_CA/1

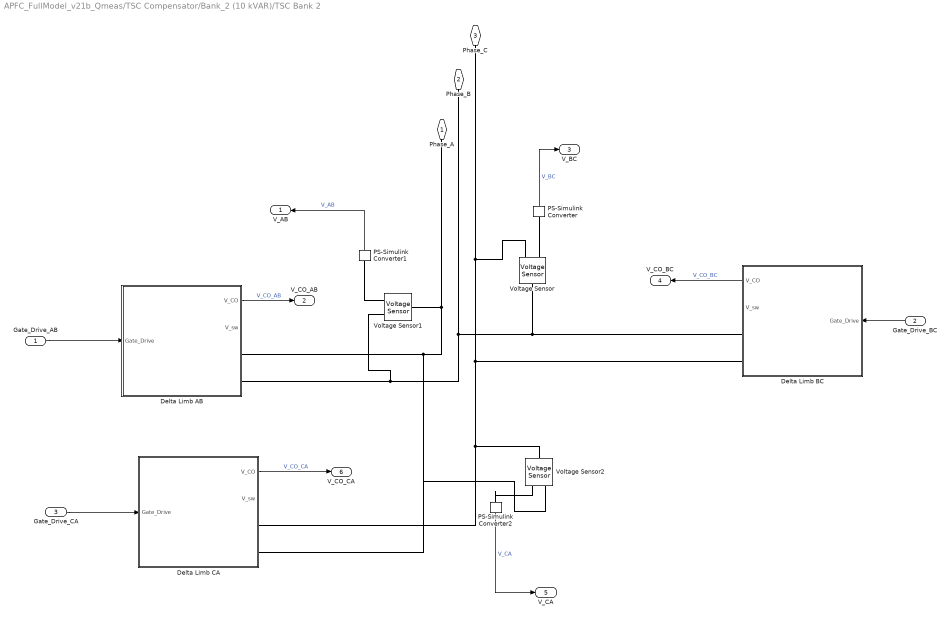
== system APFC_FullModel_v21b_Qmeas/TSC Compensator/Bank_2 (10 kVAR)/TSC Bank 2 ==
  Gate_Drive_AB : Inport
  Gate_Drive_BC : Inport  Port=2
  Gate_Drive_CA : Inport  Port=3
  Delta Limb AB : Subsystem  mask{C_val=C_B2, L_val=L_B2, Rd_val=100e3}
      mask prompts: C_val "Capacitance (F)"; L_val "Inductance (H)"; Rd_val "Discharge Resistance (Ohm)"
      mask help:
      | Delta limb of a three-phase delta-connected TSC bank.
      | Contains: anti-parallel thyristor pair, detuning reactor (L_val,
      | R_series = omega*L_val/Q_reactor), shunt capacitor (C_val), parallel discharge
      | resistor (Rd_val), RC snubber (100 Ohm, 0.1 uF).
      |
      | Output signals:
      | V_sw: instantaneous voltage across the anti-parallel thyristor pair.
      | Used as a diagnostic signal to verify transient-free switching.
      | At the moment of firing, V_sw should be at or near zero. After
      | turn-off, V_sw reflects the difference between the line-to-line
      | source voltage and the capacitor voltage V_C0.
      |
      | V_C0: instantaneous voltage across the shunt capacitor. Fed
      | externally to the ZCD comparator as the residual capacitor voltage
      | reference for voltage-matched firing on subsequent switching events.
      |
      | ZCD logic and gate drive signals are external to this subsystem.
      | Default values correspond to Bank 3 (20 kVAR) at 415 V / 50 Hz
      | with 6% detuning factor. Parameter values for Bank 1 (5 kVAR) and
      | Bank 2 (10 kVAR) are assigned by editing the mask dialog at
      | instantiation.
  Delta Limb BC : Subsystem  mask{C_val=C_B2, L_val=L_B2, Rd_val=100e3}
      mask prompts: C_val "Capacitance (F)"; L_val "Inductance (H)"; Rd_val "Discharge Resistance (Ohm)"
      mask help:
      | Delta limb of a three-phase delta-connected TSC bank.
      | Contains: anti-parallel thyristor pair, detuning reactor (L_val,
      | R_series = omega*L_val/Q_reactor), shunt capacitor (C_val), parallel discharge
      | resistor (Rd_val), RC snubber (100 Ohm, 0.1 uF).
      |
      | Output signals:
      | V_sw: instantaneous voltage across the anti-parallel thyristor pair.
      | Used as a diagnostic signal to verify transient-free switching.
      | At the moment of firing, V_sw should be at or near zero. After
      | turn-off, V_sw reflects the difference between the line-to-line
      | source voltage and the capacitor voltage V_C0.
      |
      | V_C0: instantaneous voltage across the shunt capacitor. Fed
      | externally to the ZCD comparator as the residual capacitor voltage
      | reference for voltage-matched firing on subsequent switching events.
      |
      | ZCD logic and gate drive signals are external to this subsystem.
      | Default values correspond to Bank 3 (20 kVAR) at 415 V / 50 Hz
      | with 6% detuning factor. Parameter values for Bank 1 (5 kVAR) and
      | Bank 2 (10 kVAR) are assigned by editing the mask dialog at
      | instantiation.
  Delta Limb CA : Subsystem  mask{C_val=C_B2, L_val=L_B2, Rd_val=100e3}
      mask prompts: C_val "Capacitance (F)"; L_val "Inductance (H)"; Rd_val "Discharge Resistance (Ohm)"
      mask help:
      | Delta limb of a three-phase delta-connected TSC bank.
      | Contains: anti-parallel thyristor pair, detuning reactor (L_val,
      | R_series = omega*L_val/Q_reactor), shunt capacitor (C_val), parallel discharge
      | resistor (Rd_val), RC snubber (100 Ohm, 0.1 uF).
      |
      | Output signals:
      | V_sw: instantaneous voltage across the anti-parallel thyristor pair.
      | Used as a diagnostic signal to verify transient-free switching.
      | At the moment of firing, V_sw should be at or near zero. After
      | turn-off, V_sw reflects the difference between the line-to-line
      | source voltage and the capacitor voltage V_C0.
      |
      | V_C0: instantaneous voltage across the shunt capacitor. Fed
      | externally to the ZCD comparator as the residual capacitor voltage
      | reference for voltage-matched firing on subsequent switching events.
      |
      | ZCD logic and gate drive signals are external to this subsystem.
      | Default values correspond to Bank 3 (20 kVAR) at 415 V / 50 Hz
      | with 6% detuning factor. Parameter values for Bank 1 (5 kVAR) and
      | Bank 2 (10 kVAR) are assigned by editing the mask dialog at
      | instantiation.
  PS-Simulink Converter : nesl_utility/PS-Simulink Converter  PhysicalDomain=network_engine_domain  SubClassName=ps_output  LeftPortType=input  RightPortType=output  PseudoPeriodic=off  Frequencies=[]  VectorFormat=inherit  Unit=inherit  AffineConversion=off
  PS-Simulink Converter1 : nesl_utility/PS-Simulink Converter  PhysicalDomain=network_engine_domain  SubClassName=ps_output  LeftPortType=input  RightPortType=output  PseudoPeriodic=off  Frequencies=[]  VectorFormat=inherit  Unit=inherit  AffineConversion=off
  PS-Simulink Converter2 : nesl_utility/PS-Simulink Converter  PhysicalDomain=network_engine_domain  SubClassName=ps_output  LeftPortType=input  RightPortType=output  PseudoPeriodic=off  Frequencies=[]  VectorFormat=inherit  Unit=inherit  AffineConversion=off
  Voltage Sensor : fl_lib/Electrical/Electrical Sensors/Voltage Sensor
  Voltage Sensor1 : fl_lib/Electrical/Electrical Sensors/Voltage Sensor
  Voltage Sensor2 : fl_lib/Electrical/Electrical Sensors/Voltage Sensor
  Phase_A : PMIOPort  Side=Left
  Phase_B : PMIOPort  Port=2  Side=Left
  Phase_C : PMIOPort  Port=3  Side=Left
  V_AB : Outport
  V_CO_AB : Outport  Port=2
  V_BC : Outport  Port=3
  V_CO_BC : Outport  Port=4
  V_CA : Outport  Port=5
  V_CO_CA : Outport  Port=6
  wires:
  Delta Limb BC/1(V_CO) -> V_CO_BC/1  "V_CO_BC"
  PS-Simulink Converter/1 -> V_BC/1  "V_BC"
  Gate_Drive_CA/1 -> Delta Limb CA/1(Gate_Drive)
  PS-Simulink Converter1/1 -> V_AB/1  "V_AB"
  Delta Limb AB/1(V_CO) -> V_CO_AB/1  "V_CO_AB"
  Delta Limb CA/1(V_CO) -> V_CO_CA/1  "V_CO_CA"
  Gate_Drive_BC/1 -> Delta Limb BC/1(Gate_Drive)
  Gate_Drive_AB/1 -> Delta Limb AB/1(Gate_Drive)
  PS-Simulink Converter2/1 -> V_CA/1  "V_CA"
  connections:
  Delta Limb BC/RConn1 -- Voltage Sensor/LConn1 -- Phase_B/RConn1 -- Voltage Sensor1/RConn2 -- Delta Limb AB/RConn2
  Voltage Sensor1/RConn1 -- PS-Simulink Converter1/LConn1
  PS-Simulink Converter2/LConn1 -- Voltage Sensor2/RConn1
  Voltage Sensor/RConn2 -- Phase_C/RConn1 -- Delta Limb BC/RConn2 -- Voltage Sensor2/LConn1 -- Delta Limb CA/RConn1
  Voltage Sensor/RConn1 -- PS-Simulink Converter/LConn1
  Voltage Sensor1/LConn1 -- Phase_A/RConn1 -- Voltage Sensor2/RConn2 -- Delta Limb CA/RConn2 -- Delta Limb AB/RConn1

== system APFC_FullModel_v21b_Qmeas/TSC Compensator/Bank_2 (10 kVAR)/ZCD Bank 2 ==
  V_AB : Inport
  V_CO_AB : Inport  Port=2
  V_BC : Inport  Port=3
  V_CO_BC : Inport  Port=4
  V_CA : Inport  Port=5
  V_CO_CA : Inport  Port=6
  Enable : Inport  Port=7
  ZCD AB : Subsystem
      mask help:
      | Zero-Crossing Detection (ZCD) subsystem for one delta limb of a
      | three-phase delta-connected TSC bank.
      |
      | Implements voltage-matched firing logic for transient-free
      | thyristor switching.
      |
      | Inputs:
      | V_source: instantaneous line-to-line voltage for this limb,
      | fed through a Unit Delay (T_s = 0.0001 s) to the comparator.
      |
      | V_C0: residual capacitor voltage from the corresponding
      | Delta_Limb instance, fed through a Unit Delay (T_s = 0.0001 s)
      | to the comparator.
      |
      | Enable: FLC switching command (S = 1 to arm, S = 0 to inhibit).
      | Set to Constant = 1 for open-loop testing.
      |
      | Output:
      | Gate_drive: firing pulse issued when V_source >= V_C0 on a
      | rising edge, AND Enable = 1. Fed to the Gate_drive inport of
      | the corresponding Delta_Limb instance.
      |
      | Internal blocks: Unit Delay (x2), Relational Operator (>=),
      | Zero-Order Hold (T_s = 0.0001 s), Edge Detector (rising edge),
      | AND gate.
      |
      | One instance required per delta limb: ZCD_AB, ZCD_BC, ZCD_CA.
  ZCD BC : Subsystem
      mask help:
      | Zero-Crossing Detection (ZCD) subsystem for one delta limb of a
      | three-phase delta-connected TSC bank.
      |
      | Implements voltage-matched firing logic for transient-free
      | thyristor switching.
      |
      | Inputs:
      | V_source: instantaneous line-to-line voltage for this limb,
      | fed through a Unit Delay (T_s = 0.0001 s) to the comparator.
      |
      | V_C0: residual capacitor voltage from the corresponding
      | Delta_Limb instance, fed through a Unit Delay (T_s = 0.0001 s)
      | to the comparator.
      |
      | Enable: FLC switching command (S = 1 to arm, S = 0 to inhibit).
      | Set to Constant = 1 for open-loop testing.
      |
      | Output:
      | Gate_drive: firing pulse issued when V_source >= V_C0 on a
      | rising edge, AND Enable = 1. Fed to the Gate_drive inport of
      | the corresponding Delta_Limb instance.
      |
      | Internal blocks: Unit Delay (x2), Relational Operator (>=),
      | Zero-Order Hold (T_s = 0.0001 s), Edge Detector (rising edge),
      | AND gate.
      |
      | One instance required per delta limb: ZCD_AB, ZCD_BC, ZCD_CA.
  ZCD CA : Subsystem
      mask help:
      | Zero-Crossing Detection (ZCD) subsystem for one delta limb of a
      | three-phase delta-connected TSC bank.
      |
      | Implements voltage-matched firing logic for transient-free
      | thyristor switching.
      |
      | Inputs:
      | V_source: instantaneous line-to-line voltage for this limb,
      | fed through a Unit Delay (T_s = 0.0001 s) to the comparator.
      |
      | V_C0: residual capacitor voltage from the corresponding
      | Delta_Limb instance, fed through a Unit Delay (T_s = 0.0001 s)
      | to the comparator.
      |
      | Enable: FLC switching command (S = 1 to arm, S = 0 to inhibit).
      | Set to Constant = 1 for open-loop testing.
      |
      | Output:
      | Gate_drive: firing pulse issued when V_source >= V_C0 on a
      | rising edge, AND Enable = 1. Fed to the Gate_drive inport of
      | the corresponding Delta_Limb instance.
      |
      | Internal blocks: Unit Delay (x2), Relational Operator (>=),
      | Zero-Order Hold (T_s = 0.0001 s), Edge Detector (rising edge),
      | AND gate.
      |
      | One instance required per delta limb: ZCD_AB, ZCD_BC, ZCD_CA.
  Gate_drive_AB : Outport
  Gate_drive_BC : Outport  Port=2
  Gate_drive_CA : Outport  Port=3
  wires:
  V_BC/1 -> ZCD BC/2(V_BC)
  Enable/1 -> ZCD AB/3(Enable), ZCD CA/3(Enable), ZCD BC/3(Enable)
  V_CO_BC/1 -> ZCD BC/1(V_CO_BC)
  V_CA/1 -> ZCD CA/2(V_CA)
  V_AB/1 -> ZCD AB/2(V_AB)
  ZCD BC/1(Gate_drive_BC) -> Gate_drive_BC/1
  V_CO_CA/1 -> ZCD CA/1(V_CO_CA)
  ZCD AB/1(Gate_drive_AB) -> Gate_drive_AB/1
  V_CO_AB/1 -> ZCD AB/1(V_CO_AB)
  ZCD CA/1(Gate_drive_CA) -> Gate_drive_CA/1
